simulink model "halfcar"  (R2021b)
settings: Solver=VariableStepAuto  StartTime=0.0  StopTime=10.0  RelTol=1e-3
settings Model: Creator=user  LastModifiedBy=user

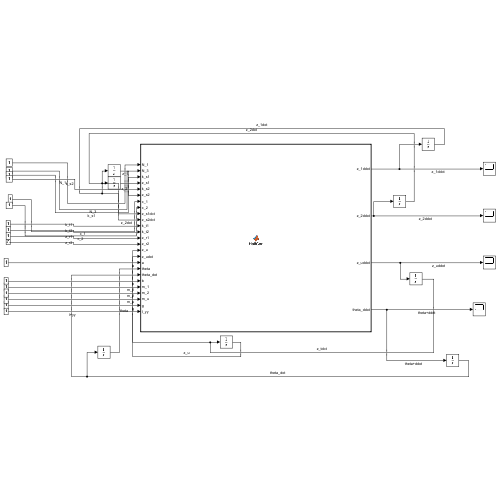
[thumbnail: Simulink's stored preview of the top-level diagram]
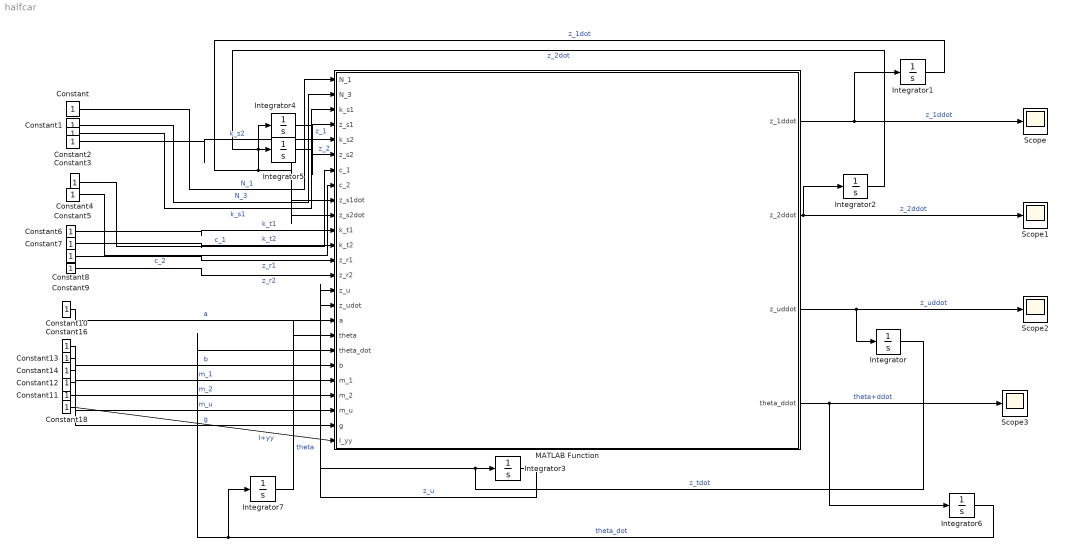
== system halfcar ==
  Constant{,1..14,16,18} (17 alike) : Constant
  Integrator{,1..7} (8 alike) : Integrator
  MATLAB Function : MATLAB Function  TreatAsAtomicUnit=on
  Scope{,1..3} (4 alike) : Scope
  wires:
  Constant/1 -> MATLAB Function/1(N_1)  "N_1"
  Constant1/1 -> MATLAB Function/2(N_3)  "N_3"
  MATLAB Function/1(z_1ddot) -> Integrator1/1, Scope/1  "z_1ddot"
  MATLAB Function/2(z_2ddot) -> Integrator2/1, Scope1/1  "z_2ddot"
  MATLAB Function/3(z_uddot) -> Integrator/1, Scope2/1  "z_uddot"
  Integrator/1 -> Integrator3/1, MATLAB Function/16(z_udot)  "z_tdot"
  Integrator1/1 -> Integrator4/1, MATLAB Function/9(z_s1dot)  "z_1dot"
  Integrator2/1 -> Integrator5/1, MATLAB Function/10(z_s2dot)  "z_2dot"
  Integrator3/1 -> MATLAB Function/15(z_u)  "z_u"
  Integrator4/1 -> MATLAB Function/4(z_s1)  "z_1"
  Integrator5/1 -> MATLAB Function/6(z_s2)  "z_2"
  Constant2/1 -> MATLAB Function/3(k_s1)  "k_s1"
  Constant3/1 -> MATLAB Function/5(k_s2)  "k_s2"
  Constant4/1 -> MATLAB Function/7(c_1)  "c_1"
  Constant5/1 -> MATLAB Function/8(c_2)  "c_2"
  Constant6/1 -> MATLAB Function/11(k_t1)  "k_t1"
  Constant7/1 -> MATLAB Function/12(k_t2)  "k_t2"
  Constant8/1 -> MATLAB Function/13(z_r1)  "z_r1"
  Constant9/1 -> MATLAB Function/14(z_r2)  "z_r2"
  Constant10/1 -> MATLAB Function/17(a)  "a"
  Constant11/1 -> MATLAB Function/24(g)  "g"
  Constant12/1 -> MATLAB Function/23(m_u)  "m_u"
  Constant13/1 -> MATLAB Function/21(m_1)  "m_1"
  Constant14/1 -> MATLAB Function/22(m_2)  "m_2"
  Constant16/1 -> MATLAB Function/20(b)  "b"
  Constant18/1 -> MATLAB Function/25(I_yy)  "I+yy"
  MATLAB Function/4(theta_ddot) -> Integrator6/1, Scope3/1  "theta+ddot"
  Integrator6/1 -> Integrator7/1, MATLAB Function/19(theta_dot)  "theta_dot"
  Integrator7/1 -> MATLAB Function/18(theta)  "theta"

== matlab function halfcar/MATLAB Function ==
  data: N_1 input; z_1ddot output; N_3 input; k_s1 input; z_s1 input; k_s2 input; z_s2 input; c_1 input; c_2 input; z_s1dot input; z_s2dot input; k_t1 input; k_t2 input; z_r1 input; z_r2 input; z_u input; z_udot input; a input; theta input; theta_dot input; b input; m_1 input; m_2 input; m_u input; g input; z_2ddot output; z_uddot output; I_yy input; theta_ddot output
function [z_1ddot, z_2ddot, z_uddot, theta_ddot] = HalfCar(N_1, N_3, k_s1, z_s1, k_s2, z_s2, c_1, c_2, z_s1dot, z_s2dot, k_t1, k_t2, z_r1, z_r2, z_u, z_udot, a, theta,  theta_dot, b, m_1, m_2, m_u, g, I_yy)
    z_1ddot = (N_1 - m_1 .* g - (k_s1 .* z_s1 + c_1 .* z_s1dot) - k_t1 .* (z_s1 - z_r1) + k_s1 .* z_u + c_1 .* z_udot - k_s1 .* (a .* theta) - c_1 .* (a .*theta_dot) / m_1
    z_2ddot = (N_3 - m_2 .* g - (k_s2 .* z_s2 + c_2 .* z_s2dot) - k_t2 .* (z_s2 - z_r2) + k_s2 .* z_u + c_2 .* z_udot + k_s2 .* (b .* theta) + c_2 .* (b .* theta_dot)) / m_2
    z_uddot = (k_s1 .* z_s1 + c_1 .* z_s1dot + k_s2 .* z_s2 + c_2 .* z_s2dot - (k_s1 .* z_u + c_1 .* z_udot) - (k_s2 .* z_u + c_2 .* z_udot) + k_s1 .* (a .* theta) +c_1 .* (a .*theta_dot) - k_s2 .* (b .* theta) - c_2 .* (b .* theta_dot)) / m_u
    theta_ddot = (-a .* (k_s1 .* z_s1 + c_1 .* z_s1dot - k_s1 .* z_u - c_1 .* z_udot + k_s1 .* (a .* theta) + c_1 .* (a .* theta_dot) + b .* (k_s2 .* z_s2 + c_2 .* z_s2dot - k_s2 .* z_u - c_2 .* z_udot - k_s2 .* (b .* theta) - c_2 .* (b .* theta_dot))) / I_yy
end
